simulink model "EV_RigidShaft"  (R2026a)
settings: Solver=ode45  StopTime=StepStopTime  MaxStep=MaxStep  RelTol=RelTol  AbsTol=AbsTol
values from neighbouring files (symbols this model uses):
  Ip = 1    [RigidShaft_parameters.m]
  k = 10    [RigidShaft_parameters.m]
  L = 1    [RigidShaft_parameters.m]
  R = 1    [RigidShaft_parameters.m]
  t_step_M = 0.8    [RigidShaft_parameters.m]
  t_step_V = 0.1    [RigidShaft_parameters.m]
settings Model: Creator=dinul  LastModifiedBy=dinul

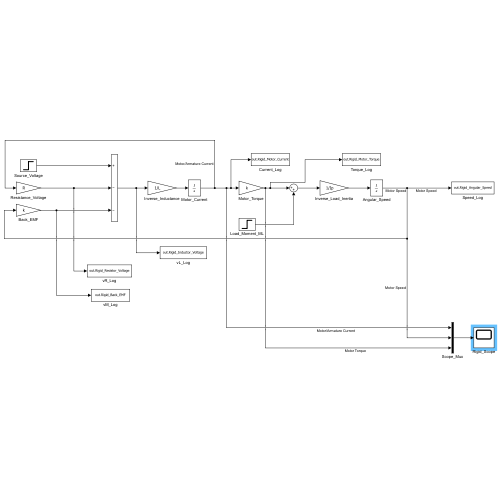
[thumbnail: Simulink's stored preview of the top-level diagram]
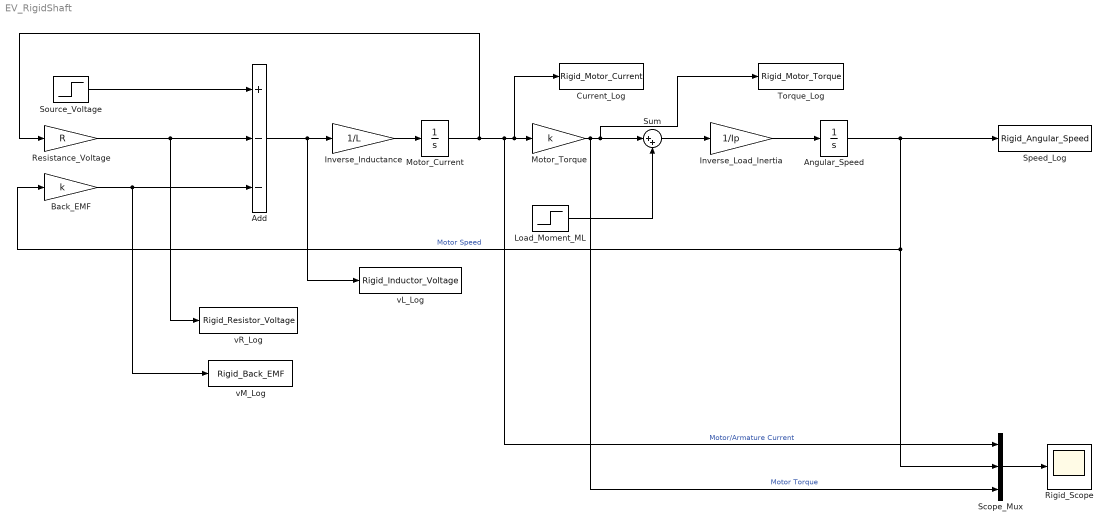
== system EV_RigidShaft ==
  Add : Sum  Inputs=+--
  Angular_Speed : Integrator
  Back_EMF : Gain  Gain=k
  Current_Log : ToWorkspace  VariableName=Rigid_Motor_Current  SaveFormat=Timeseries  SampleTime=-1
  Inverse_Inductance : Gain  Gain=1/L
  Inverse_Load_Inertia : Gain  Gain=1/Ip
  Load_Moment_ML : Step  Time=t_step_M  FinalValue=ML_model_amp  SampleTime=0
  Motor_Current : Integrator
  Motor_Torque : Gain  Gain=k
  Resistance_Voltage : Gain  Gain=R
  Rigid_Scope : Scope
  Scope_Mux : Mux  Inputs=3
  Source_Voltage : Step  Time=t_step_V  FinalValue=Vs_step_amp  SampleTime=0
  Speed_Log : ToWorkspace  VariableName=Rigid_Angular_Speed  SaveFormat=Timeseries  SampleTime=-1
  Sum : Sum  Inputs=|++
  Torque_Log : ToWorkspace  VariableName=Rigid_Motor_Torque  SaveFormat=Timeseries  SampleTime=-1
  vL_Log : ToWorkspace  VariableName=Rigid_Inductor_Voltage  SaveFormat=Timeseries  SampleTime=-1
  vM_Log : ToWorkspace  VariableName=Rigid_Back_EMF  SaveFormat=Timeseries  SampleTime=-1
  vR_Log : ToWorkspace  VariableName=Rigid_Resistor_Voltage  SaveFormat=Timeseries  SampleTime=-1
  wires:
  Source_Voltage/1 -> Add/1
  Add/1 -> Inverse_Inductance/1, vL_Log/1
  Inverse_Inductance/1 -> Motor_Current/1
  Motor_Current/1 -> Motor_Torque/1, Current_Log/1, Scope_Mux/1, Resistance_Voltage/1  "Motor/Armature Current"
  Resistance_Voltage/1 -> Add/2, vR_Log/1
  Angular_Speed/1 -> Back_EMF/1, Scope_Mux/2, Speed_Log/1  "Motor Speed"
  Back_EMF/1 -> Add/3, vM_Log/1
  Motor_Torque/1 -> Torque_Log/1, Sum/1, Scope_Mux/3  "Motor Torque"
  Load_Moment_ML/1 -> Sum/2
  Sum/1 -> Inverse_Load_Inertia/1
  Inverse_Load_Inertia/1 -> Angular_Speed/1
  Scope_Mux/1 -> Rigid_Scope/1
